simulink model "DiscreteBuck_Offline_Control4"  (R2025a)
settings: Solver=FixedStepDiscrete  StartTime=0.0  StopTime=SimTime  FixedStep=Tsim  RelTol=1e-9
undefined symbols (not defined in the file): C_buck, DiscIntNeverNeededParam, Iout_buck, kd, ki, kp, L_buck, R, Tsim, Tsw, Vg, Vout_buck
libraries: slpidlib x1, spsPWMGeneratorDCDCLib x1
settings Model: Creator=Andres  LastModifiedBy=Andres
settings DataIOCC: ReturnWorkspaceOutputs=off  SignalLoggingName=ResultDisc

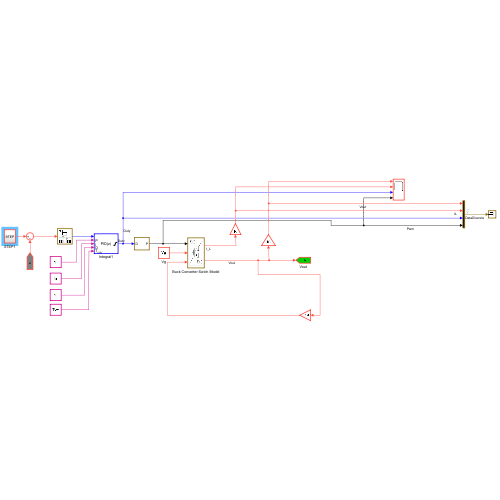
[thumbnail: Simulink's stored preview of the top-level diagram]
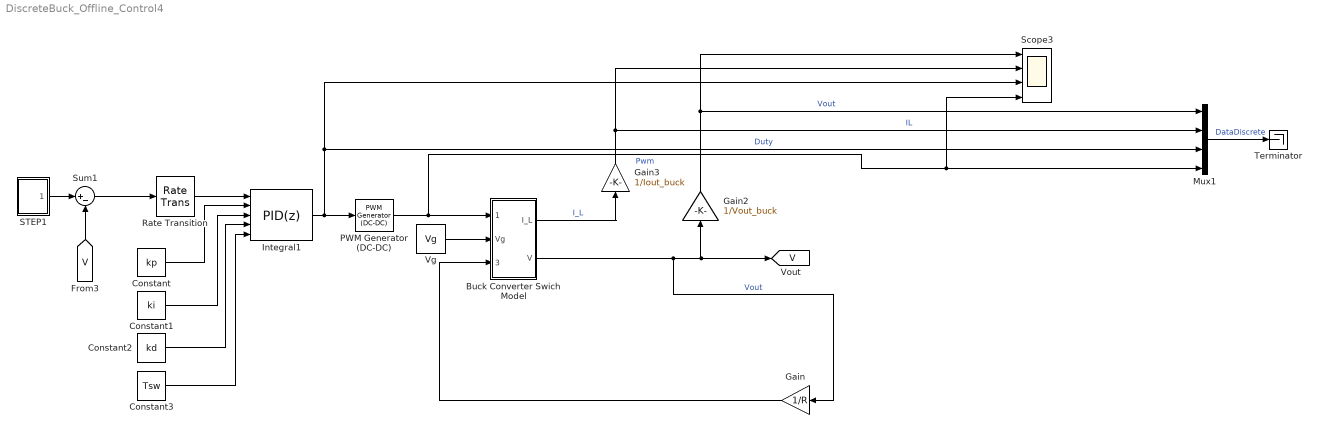
== system DiscreteBuck_Offline_Control4 ==
  Buck Converter Swich Model : Subsystem
      mask Display: image('$imagefile'); % Use "Edit Image" on toolstrip to change.
  Constant : Constant  Value=kp
  Constant1 : Constant  Value=ki
  Constant2 : Constant  Value=kd
  Constant3 : Constant  Value=Tsw
  Gain : Gain  Gain=1/R
  Gain2 : Gain  Gain=1/Vout_buck
  Gain3 : Gain  Gain=1/Iout_buck
  Integral1 : slpidlib/PID Controller  Controller=PID  Form=Parallel  TimeDomain=Discrete-time  UseExternalTs=on  SampleTime=Tsw  IntegratorMethod=Trapezoidal  FilterMethod=Forward Euler  ControllerParametersSource=external  P=kp  I=ki  UseKiTs=off  D=kd  UseExternalDerivativeSource=off  N=1  UseFilter=off  TunerSelectOption=Transfer Function Based (PID Tuner App)  InitialConditionSource=internal  InitialConditionForIntegrator=0  InitialConditionForFilter=0  DifferentiatorICPrevScaledInput=0  ExternalReset=none  IgnoreLimit=on  TrackingMode=off  Kt=1  LimitOutput=on  SatLimitsSource=internal  UpperSaturationLimit=0.98  LowerSaturationLimit=0  LinearizeAsGain=on  AntiWindupMode=clamping  Kb=1  LimitIntegrator=off  UpperIntegratorSaturationLimit=inf  LowerIntegratorSaturationLimit=-inf  POutMin=[]  POutMax=[]  IOutMin=[]  IOutMax=[]  DOutMin=[]  DOutMax=[]  NOutMin=[]  NOutMax=[]  SumOutMin=[]  SumOutMax=[]  SaturationOutMin=[]  SaturationOutMax=[]  PParamMin=[]  PParamMax=[]  IParamMin=[]  IParamMax=[]  DParamMin=[]  DParamMax=[]  NParamMin=[]  NParamMax=[]  KbParamMin=[]  KbParamMax=[]  KtParamMin=[]  KtParamMax=[]  KbOutMin=[]  KbOutMax=[]  KtOutMin=[]  KtOutMax=[]  IntegratorOutMin=[]  IntegratorOutMax=[]  FilterOutMin=[]  FilterOutMax=[]  SumI1OutMin=[]  SumI1OutMax=[]  SumI2OutMin=[]  SumI2OutMax=[]  SumI3OutMin=[]  SumI3OutMax=[]  SumI4OutMin=[]  SumI4OutMax=[]  SumDOutMin=[]  SumDOutMax=[]  DifferentiatorOutMin=[]  DifferentiatorOutMax=[]  FilterDiffOutCoefMin=[]  FilterDiffOutCoefMax=[]  ReciprocalOutMin=[]  ReciprocalOutMax=[]  SumDenOutMin=[]  SumDenOutMax=[]  SumNumOutMin=[]  SumNumOutMax=[]  DivideOutMin=[]  DivideOutMax=[]  UdiffTsProdOutMin=[]  UdiffTsProdOutMax=[]  NTsProdOutMin=[]  NTsProdOutMax=[]  UintegralTsProdOutMin=[]  UintegralTsProdOutMax=[]  UngainTsProdOutMin=[]  UngainTsProdOutMax=[]  ClampingZeroOutDataTypeStr=Inherit: Inherit via back propagation  ClampingZeroOutMin=[]  ClampingZeroOutMax=[]  FilterDenConstantOutDataTypeStr=Inherit: Inherit via back propagation  FilterDenConstantOutMin=[]  FilterDenConstantOutMax=[]  PCopyOutDataTypeStr=Inherit: Inherit via back propagation  PCopyOutMin=[]  PCopyOutMax=[]  NCopyOutDataTypeStr=Inherit: Inherit via back propagation  NCopyOutMin=[]  NCopyOutMax=[]  IntegratorContinuousStateAttributes=''  IntegratorStateMustResolveToSignalObject=off  IntegratorRTWStateStorageClass=Auto  FilterContinuousStateAttributes=''  FilterStateMustResolveToSignalObject=off  FilterRTWStateStorageClass=Auto  ParallelPVariant=ExternalParameters  IdealPVariant=Disabled  IVariant=ExternalParameters  DVariant=ExternalParameters  IntegratorVariant=Discrete  SatVariant=Enabled  AWVariant=DiscClampingParallel  PCopyVariant=Disabled  TRVariant=Disabled  FdbkBlocksVariant=Feedback  IdealPFdbkVariant=Passthrough  SatFdbkVariant=Passthrough  DerivativeFilterVariant=Differentiator  NVariant=Passthrough  NCopyVariant=Disabled_SignalSpec  FilterICVariant=InternalICsDifferentiator  IntegratorICVariant=InternalICs  ExternalResetVariant=Disabled  TRSumVariant=Passthrough  SumFdbkVariant=Enabled  SumVariant=Sum_PID  TsampFilterVariant=ExternalTs  TsampNgainVariant=Passthrough  TsampIntegralVariant=ExternalTs  ExternalSaturationOutDataTypeStr=Inherit: Same as second input  DerivativeSourceVariant=ErrorSignal  PreIntVariant=InternalPreInt
  Mux1 : Mux
  PWM Generator (DC-DC) : spsPWMGeneratorDCDCLib/PWM Generator (DC-DC)  Fsw=f_sw  Ts=0
  Rate Transition : RateTransition  OutPortSampleTime=Tsw
  STEP1 : Subsystem
  Scope3 : Scope  NumInputPorts=4
      settings: ActiveDisplayString=4  ActiveDisplayYMinimum=-0.32713817832644732  ActiveDisplayYMaximum=2.9442436049380265  YLabel=Power
  Sum1 : Sum  Inputs=|+-
  Terminator : Terminator
  Vg : Constant  Value=Vg  SampleTime=-1
  tag scope: V=global
  wires:
  Vg/1 -> Buck Converter Swich Model/2(Vg)
  PWM Generator (DC-DC)/1 -> Scope3/4, Mux1/4, Buck Converter Swich Model/1(PWM)  "Pwm"
  STEP1/1(STEP) -> Sum1/1
  [V] -> Sum1/2
  Sum1/1 -> Rate Transition/1
  Buck Converter Swich Model/2(V) -> Gain2/1, [V], Gain/1  "Vout"
  Mux1/1 -> Terminator/1  "DataDiscrete"
  Integral1/1 -> Scope3/3, Mux1/3, PWM Generator (DC-DC)/1  "Duty"
  Buck Converter Swich Model/1(I_L) -> Gain3/1  "I_L"
  Rate Transition/1 -> Integral1/1
  Gain/1 -> Buck Converter Swich Model/3(I_load)
  Gain2/1 -> Scope3/1, Mux1/1  "Vout"
  Gain3/1 -> Scope3/2, Mux1/2  "IL"
  Constant/1 -> Integral1/2
  Constant1/1 -> Integral1/3
  Constant2/1 -> Integral1/4
  Constant3/1 -> Integral1/5

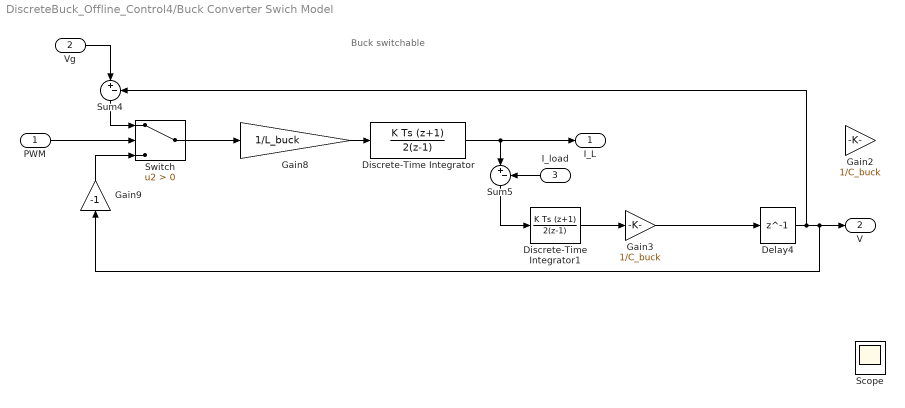
== system DiscreteBuck_Offline_Control4/Buck Converter Swich Model ==
  note: Buck switchable
  PWM : Inport
  Vg : Inport  Port=2
  I_load : Inport  Port=3
  Delay4 : Delay  DelayLength=1  InputProcessing=Columns as channels (frame based)
  Discrete-Time Integrator : DiscreteIntegrator  IntegratorMethod=Integration: Trapezoidal  SampleTime=Tsim  LimitOutput=on  LowerSaturationLimit=0  ICPrevOutput=DiscIntNeverNeededParam  ICPrevScaledInput=DiscIntNeverNeededParam
  Discrete-Time Integrator1 : DiscreteIntegrator  IntegratorMethod=Integration: Trapezoidal  SampleTime=Tsim  ICPrevOutput=DiscIntNeverNeededParam  ICPrevScaledInput=DiscIntNeverNeededParam
  Gain2 : Gain  Gain=1/C_buck
  Gain3 : Gain  Gain=1/C_buck
  Gain8 : Gain  Gain=1/L_buck
  Gain9 : Gain  Gain=-1
  Scope : Scope  NumInputPorts=2
      settings: ActiveDisplayYMinimum=-2.4027986803455188  ActiveDisplayYMaximum=21.625188123109673
  Sum4 : Sum  Inputs=|+-
  Sum5 : Sum  Inputs=|+-
  Switch : Switch  Criteria=u2 > Threshold  SaturateOnIntegerOverflow=off  InputSameDT=off
  I_L : Outport
  V : Outport  Port=2
  wires:
  Gain9/1 -> Switch/3
  Switch/1 -> Gain8/1
  Sum4/1 -> Switch/1
  Gain8/1 -> Discrete-Time Integrator/1
  Sum5/1 -> Discrete-Time Integrator1/1
  Discrete-Time Integrator/1 -> I_L/1, Sum5/1
  Vg/1 -> Sum4/1
  I_load/1 -> Sum5/2
  PWM/1 -> Switch/2
  Delay4/1 -> Sum4/2, Gain9/1, V/1
  Discrete-Time Integrator1/1 -> Gain3/1
  Gain3/1 -> Delay4/1

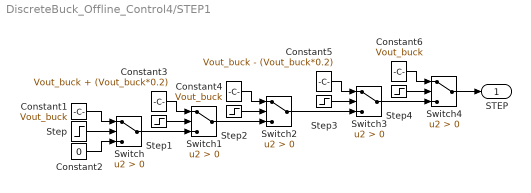
== system DiscreteBuck_Offline_Control4/STEP1 ==
  Constant1 : Constant  Value=Vout_buck  SampleTime=-1
  Constant2 : Constant  Value=0  SampleTime=-1
  Constant3 : Constant  Value=Vout_buck + (Vout_buck*0.2)  SampleTime=-1
  Constant4 : Constant  Value=Vout_buck  SampleTime=-1
  Constant5 : Constant  Value=Vout_buck - (Vout_buck*0.2)  SampleTime=-1
  Constant6 : Constant  Value=Vout_buck  SampleTime=-1
  Step : Step  Time=0.01
  Step1 : Step  Time=0.02
  Step2 : Step  Time=0.03
  Step3 : Step  Time=0.04
  Step4 : Step  Time=0.05
  Switch{,1..4} (5 alike) : Switch  Criteria=u2 > Threshold  SaturateOnIntegerOverflow=off  InputSameDT=off
  STEP : Outport
  wires:
  Step/1 -> Switch/2
  Constant3/1 -> Switch1/1
  Constant1/1 -> Switch/1
  Switch/1 -> Switch1/3
  Step1/1 -> Switch1/2
  Constant2/1 -> Switch/3
  Switch1/1 -> Switch2/3
  Step2/1 -> Switch2/2
  Constant4/1 -> Switch2/1
  Constant5/1 -> Switch3/1
  Switch2/1 -> Switch3/3
  Step3/1 -> Switch3/2
  Constant6/1 -> Switch4/1
  Switch3/1 -> Switch4/3
  Step4/1 -> Switch4/2
  Switch4/1 -> STEP/1
